simulink model "QuarterCarModel"  (R2021b)
settings: Solver=VariableStepAuto  StartTime=0.0  StopTime=10.0  RelTol=1e-3
undefined symbols (not defined in the file or in its folder): sigbuilder_block
settings Model: Creator=joems  LastModifiedBy=jpchi
settings SolverCC: AlgebraicLoopSolver=TrustRegion
settings DebuggingCC: SFMachineParentedDataDiag=warning

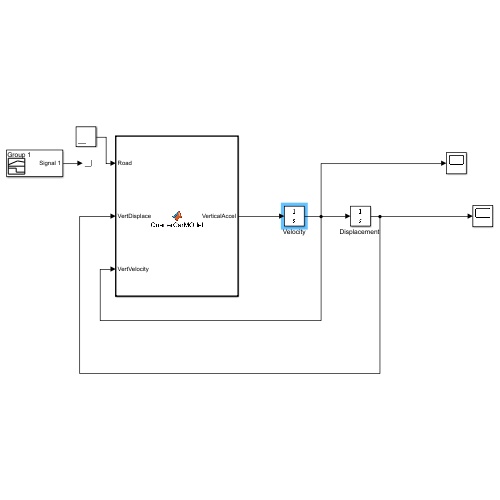
[thumbnail: Simulink's stored preview of the top-level diagram]
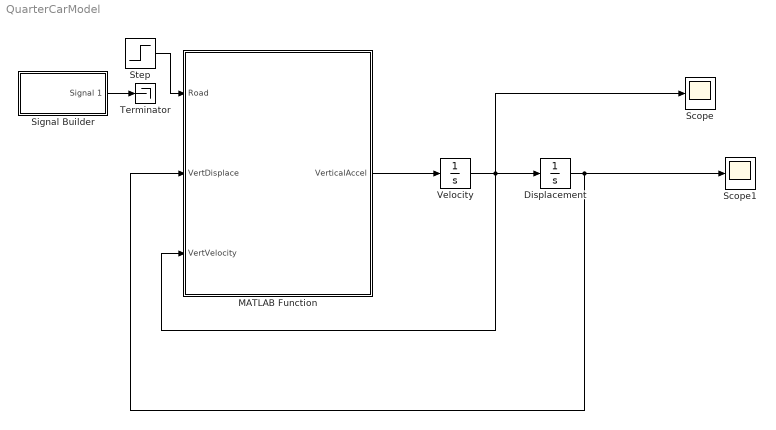
== system QuarterCarModel ==
  "Displacement " : Integrator  InitialCondition=[4,9]
  MATLAB Function : MATLAB Function  TreatAsAtomicUnit=on
  Scope : Scope
  Scope1 : Scope
  Signal Builder : Subsystem  Tag=STV Subsys  LoadFcn=sigbuilder_block('load');  StartFcn=sigbuilder_block('start');  StopFcn=sigbuilder_block('stop');  ClipboardFcn=sigbuilder_block('clipboard');  mask(Sigbuilder block){tuvar=[0:10]}
      mask help: Simulink:masks:SigbuilderBlock_MD
      mask init:
      | if ~strcmp(get_param(bdroot(gcbh),'SimulationStatus'),'stopped') tuvar = sigbuilder_block('maskInit'); end
      settings: CopyFcn=sigbuilder_block('copy');  DeleteFcn=sigbuilder_block('delete');  ModelCloseFcn=sigbuilder_block('modelClose');  PreSaveFcn=sigbuilder_block('preSave');  PauseFcn=sigbuilder_block('pause');  ContinueFcn=sigbuilder_block('continue');  NameChangeFcn=sigbuilder_block('namechange');  OpenFcn=sigbuilder_block('open',[437.6 199.2 550.4 400 ]);  CloseFcn=sigbuilder_block('close');
      mask Display: plot(0, 0, 100, 100,[2, 2, 32, 32, 2], [68, 8, 8, 68, 68],[32, 2], [38, 38], [32, 19, 2],[53, 60, 44], [32, 17, 17, 2],[16, 16, 31, 31]);txt = getActiveGroup(gcbh);text(2, 100, txt,'verticalAlignment', 'top');
  Step : Step  Time=3  After=.1  SampleTime=0
  Terminator : Terminator
  Velocity : Integrator  InitialCondition=[2,5]
  wires:
  MATLAB Function/1(VerticalAccel) -> Velocity/1
  Velocity/1 -> Scope/1, MATLAB Function/3(VertVelocity), "Displacement "/1
  "Displacement "/1 -> Scope1/1, MATLAB Function/2(VertDisplace)
  Signal Builder/1(Signal 1) -> Terminator/1
  Step/1 -> MATLAB Function/1(Road)

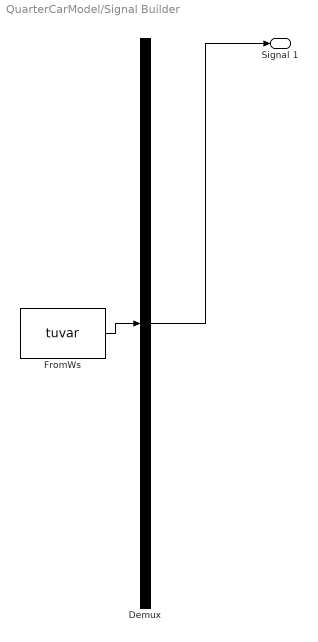
== system QuarterCarModel/Signal Builder ==
  Demux : Demux  Tag=STV Demux  Outputs=1
      settings: DisplayOption=none
  FromWs : FromWorkspace  Tag=STV FromWs  VariableName=tuvar
      SigBuilderData=|
      | common.afterFinalStr = 'Extrapolate'
      | common.sampleTime = 0
      | dataSet.timeRange = [0 10]
      | dataSet.name = 'Group 1'
      | sbobj.Groups.Name = 'Group 1'
      | sbobj.Groups.Signals.Name = 'Signal 1'
      | sbobj.Groups.Signals.XData = [0 4 6 10]
      | sbobj.Groups.Signals.YData = [0 0.005 0.99 0.99]
  Signal 1 : Outport  Tag=STV Outport
  wires:
  Demux/1 -> Signal 1/1
  FromWs/1 -> Demux/1

== matlab function QuarterCarModel/MATLAB Function ==
  data: VerticalAccel output; Road input; Parameter parameter; VertDisplace input; VertVelocity input
function VerticalAccel= QuarterCarMOdel(Road, Parameter, VertDisplace,VertVelocity )



%% Acceleration Calculation 

UnsprungVertAccel = (Parameter.SuspensionSpringStiff.*(VertDisplace(2) - VertDisplace(1))...
    + Parameter.DampingCoeff.*(VertVelocity(2) - VertVelocity(1)) ...
    - Parameter.TireStiff.*(VertDisplace(1) - Road))./Parameter.UnsprungMass;
SrungVertAccel = (-Parameter.SuspensionSpringStiff.*(VertDisplace(2) - VertDisplace(1))...
    - Parameter.DampingCoeff.*(VertVelocity(2) - VertVelocity(1)))./Parameter.SprungMass;

VerticalAccel = [UnsprungVertAccel;SrungVertAccel];
end
